simulink model "Observadores_Mimo19"  (R2023b)
settings: Solver=ode23t  StartTime=0.0  StopTime=5  MaxStep=1e-3  RelTol=1e-3
values from neighbouring files (symbols this model uses):
  Ac = reg.a    [Observdores_funcion_lqg.m]    (also in Observdores_pto_equilibrio.m)
  Ac_1 = [AL-BL*Kest-L*CL+L*DL*Kest, BL*Ki - L*DL*Ki ... (first row only)    [Observdores.m]
  Ac_2 = reg.a    [Observdores.m]    (also in Observdores_funcion_lqg.m; lqg_funcion.m)
  AL = double(subs(A,{a,b,c,d},{a1,b1,c1,d1}))    [Observdores.m]    (also in Observdores_funcion_lqg.m = double(subs(A,{x1,x2,x3,x4,u1,u2,u3,u4},{x10,x20,x30,x40,u10; Observdores_pto_equilibrio.m; Observdores_pto_equilibrio_discreto.m; Observdores_seguimiento_discreto.m)
  Bc = reg.b    [Observdores_funcion_lqg.m]    (also in Observdores_pto_equilibrio.m)
  Bc_1 = [-L ... (first row only)    [Observdores.m]
  Bc_2 = reg.b    [Observdores.m]    (also in Observdores_funcion_lqg.m; lqg_funcion.m)
  BL = double(subs(B,{a,b,c,d},{a1,b1,c1,d1}))    [Observdores.m]    (also in Observdores_funcion_lqg.m = double(subs(B,{x1,x2,x3,x4,u1,u2,u3,u4},{x10,x20,x30,x40,u10; Observdores_pto_equilibrio.m; Observdores_pto_equilibrio_discreto.m; Observdores_seguimiento_discreto.m)
  Cc = sys_d2.c    [Observdores.m]    (also in Observdores_funcion_lqg.m = reg.c; Observdores_pto_equilibrio.m = reg.c; Observdores_pto_equilibrio_discreto.m = -K)
  Cc_1 = [-Kest, Ki]    [Observdores.m]
  Cc_2 = reg.c    [Observdores.m]    (also in Observdores_funcion_lqg.m; lqg_funcion.m)
  Ccon = [-Kest Ki]    [Observdores_seguimiento_discreto.m]
  CL = [1 0 0 ... (first row only)    [Observdores.m]    (also in Observdores_funcion_lqg.m = [1 1 0 0; Observdores_pto_equilibrio.m; Observdores_pto_equilibrio_discreto.m; Observdores_seguimiento_discreto.m)
  Dc = reg.d    [Observdores_funcion_lqg.m]    (also in Observdores_pto_equilibrio.m; Observdores_pto_equilibrio_discreto.m = zeros(p,r))
  Dc_1 = zeros(p,r)    [Observdores.m]
  Dc_2 = reg.d    [Observdores.m]    (also in Observdores_funcion_lqg.m; lqg_funcion.m)
  Dcon = zeros(p,2*r)    [Observdores_seguimiento_discreto.m]
  DL = [0 0 0 ... (first row only)    [Observdores.m]    (also in Observdores_funcion_lqg.m = [0 0 0 0; Observdores_pto_equilibrio.m; Observdores_pto_equilibrio_discreto.m; Observdores_seguimiento_discreto.m)
  Gc = sys_d2.a    [Observdores.m]    (also in Observdores_pto_equilibrio.m = sys_c_dig.a; Observdores_pto_equilibrio_discreto.m = GL-HL*K-L*CL+L*DL*K)
  Gcon = [GL-HL*Kest-L*CL+L*DL*Kest, HL*Ki - L*DL*Ki ... (first row only)    [Observdores_seguimiento_discreto.m]
  GL = sysd.a    [Observdores_pto_equilibrio_discreto.m]    (also in Observdores_seguimiento_discreto.m)
  Hc = sys_c_dig.b    [Observdores_pto_equilibrio.m]    (also in Observdores_pto_equilibrio_discreto.m = L)
  Hcon = [zeros(n,r), L ... (first row only)    [Observdores_seguimiento_discreto.m]
  HL = sysd.b    [Observdores_pto_equilibrio_discreto.m]    (also in Observdores_seguimiento_discreto.m)
  K = place(Ahat,Bhat,delta)    [Observdores.m]
  Kest = K(:,1:n)    [Observdores.m]    (also in Observdores_seguimiento_discreto.m)
  Ki = -K(:,n+1:end)    [Observdores.m]    (also in Observdores_seguimiento_discreto.m)
  L = (place(AL',CL',delta))'    [Observdores.m]    (also in Observdores_pto_equilibrio.m; Observdores_pto_equilibrio_discreto.m = place(GL',CL',pol_obv_d)'; Observdores_seguimiento_discreto.m = place(GL',CL',pol_obv_d)')
  sys_d1 = c2d(sys_c1,Tm)    [Observdores.m]
  sys_d2 = c2d(sys_c2,Tm)    [Observdores.m]
  Tm = 0.02    [Observdores.m]    (also in Observdores_pto_equilibrio.m; Observdores_pto_equilibrio_discreto.m = 0.05; Observdores_seguimiento_discreto.m = 0.05)
  u10 = (a1*x20 + b1*x10^2)/u20    [Observdores.m]    (also in Observdores_funcion_lqg.m = 1; Observdores_pto_equilibrio.m; Observdores_pto_equilibrio_discreto.m; Observdores_seguimiento_discreto.m)
  u20 = sqrt(c1*x30*x20)    [Observdores.m]    (also in Observdores_funcion_lqg.m = sqrt(x30*x20); Observdores_pto_equilibrio.m; Observdores_pto_equilibrio_discreto.m; Observdores_seguimiento_discreto.m)
  u30 = (d1*x30 - u10)/x10    [Observdores.m]    (also in Observdores_funcion_lqg.m = (x20 + x10^2 - u20^2)/u10; Observdores_pto_equilibrio.m; Observdores_pto_equilibrio_discreto.m; Observdores_seguimiento_discreto.m)
  x10 = 2    [Observdores.m]    (also in Observdores_funcion_lqg.m; Observdores_pto_equilibrio.m; Observdores_pto_equilibrio_discreto.m; Observdores_seguimiento_discreto.m)
  x20 = 4    [Observdores.m]    (also in Observdores_funcion_lqg.m = 8; Observdores_pto_equilibrio.m; Observdores_pto_equilibrio_discreto.m; Observdores_seguimiento_discreto.m)
  x30 = 4    [Observdores.m]    (also in Observdores_funcion_lqg.m = 2; Observdores_pto_equilibrio.m; Observdores_pto_equilibrio_discreto.m; Observdores_seguimiento_discreto.m)
  xini = [0.5; -0.3; -0.7; 0.9]    [Observdores_funcion_lqg.m]    (also in Observdores_pto_equilibrio.m = [0.2; -0.3; -0.4]; Observdores_pto_equilibrio_discreto.m = [0.2; -0.3; -0.4])
undefined symbols (not defined in the file or in its folder): magnitude
libraries: simulink x22
(part 1 of 3)
settings Model: Creator=B12
settings SolverCC: AlgebraicLoopSolver=TrustRegion
settings DataIOCC: ReturnWorkspaceOutputs=off
settings DebuggingCC: UnconnectedInputMsg=warning  UnconnectedOutputMsg=warning  UnconnectedLineMsg=warning  ArithmeticOperatorsInVariantConditions=warning
settings ModelReferenceCC: EnableRefExpFcnMdlSchedulingChecks=on
settings SFSimCC: CustomCodeUndefinedFunction=UseInterfaceOnly

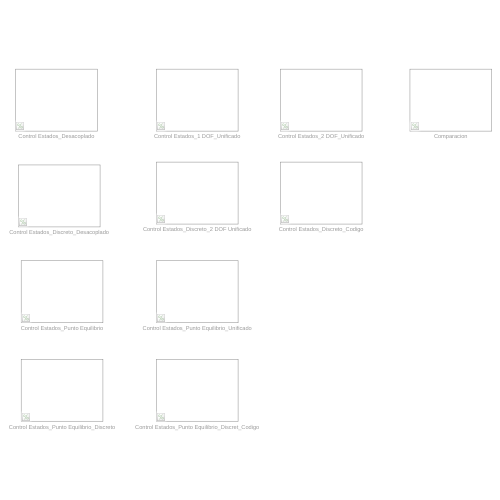
[thumbnail: Simulink's stored preview of the top-level diagram]
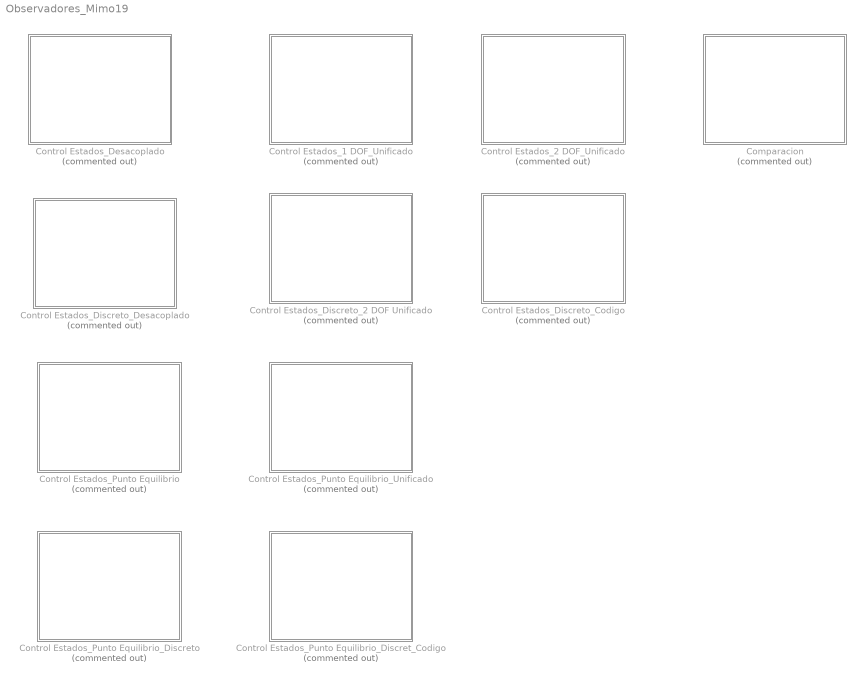
== system Observadores_Mimo19 ==
  Comparacion : Subsystem  Commented=on
  Control Estados_1 DOF_Unificado : Subsystem  Commented=on
  Control Estados_2 DOF_Unificado : Subsystem  Commented=on
  Control Estados_Desacoplado : Subsystem  Commented=on
  Control Estados_Discreto_2 DOF Unificado : Subsystem  Commented=on
  Control Estados_Discreto_Codigo : Subsystem  Commented=on
  Control Estados_Discreto_Desacoplado : Subsystem  Commented=on
  Control Estados_Punto Equilibrio : Subsystem  Commented=on
  Control Estados_Punto Equilibrio_Discret_Codigo : Subsystem  Commented=on
  Control Estados_Punto Equilibrio_Discreto : Subsystem  Commented=on
  Control Estados_Punto Equilibrio_Unificado : Subsystem  Commented=on

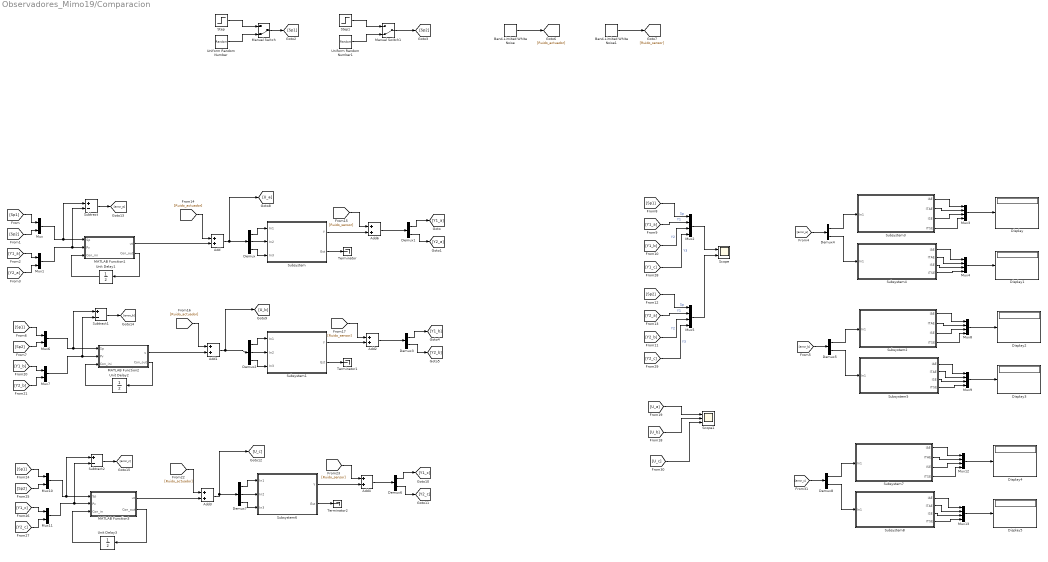
== system Observadores_Mimo19/Comparacion ==
  Add{,1..4,6} (6 alike) : Sum
  Band-Limited White Noise : simulink/Sources/Band-Limited White Noise  Cov=[1e-10 1e-10 1e-10 ]  Ts=0.001  seed=[23341]
  Band-Limited White Noise1 : simulink/Sources/Band-Limited White Noise  Cov=[1e-10 1e-10 ]  Ts=0.001  seed=[23341]
  Demux : Demux  Outputs=3
  Demux{1,3..6,8} (6 alike) : Demux  Outputs=2
  Demux2 : Demux  Outputs=3
  Demux7 : Demux  Outputs=3
  Display{,1..5} (6 alike) : Display
  MATLAB Function1 : MATLAB Function  TreatAsAtomicUnit=on
  MATLAB Function2 : MATLAB Function  TreatAsAtomicUnit=on
  MATLAB Function3 : MATLAB Function  TreatAsAtomicUnit=on
  Manual Switch : ManualSwitch  CurrentSetting=0
  Manual Switch1 : ManualSwitch  CurrentSetting=0
  Mux{,1,6..7,10..11} (6 alike) : Mux  Inputs=2
  Mux{2..5,8..9,12..13} (8 alike) : Mux
  Scope : Scope  NumInputPorts=2
  Scope1 : Scope  NumInputPorts=3
  Step : Step  Time=0  After=0.5  SampleTime=0
  Step1 : Step  Time=0  After=0.5  SampleTime=0
  Subsystem : Subsystem
  Subsystem1 : Subsystem
  Subsystem2 : Subsystem
  Subsystem3 : Subsystem
  Subsystem4 : Subsystem
  Subsystem5 : Subsystem
  Subsystem6 : Subsystem
  Subsystem7 : Subsystem
  Subsystem8 : Subsystem
  Subtract : Sum  Inputs=+-
  Subtract1 : Sum  Inputs=+-
  Subtract2 : Sum  Inputs=+-
  Terminator : Terminator
  Terminator1 : Terminator
  Terminator2 : Terminator
  Uniform Random Number : UniformRandomNumber  Minimum=-0.5  Maximum=0.5  SampleTime=4
  Uniform Random Number1 : UniformRandomNumber  Minimum=-0.5  Maximum=0.5  Seed=6  SampleTime=7
  Unit Delay1 : UnitDelay  InitialCondition=zeros(8,1)  SampleTime=Tm  HasFrameUpgradeWarning=on
  Unit Delay2 : UnitDelay  InitialCondition=zeros(8,1)  SampleTime=Tm  HasFrameUpgradeWarning=on
  Unit Delay3 : UnitDelay  InitialCondition=zeros(8,1)  SampleTime=Tm  HasFrameUpgradeWarning=on
  wires:
  [Sp2] -> Mux5/1  "Sp"
  [Y1_a] -> Mux2/2  "Y1"
  [U_a] -> Scope1/1
  [Y2_a] -> Mux5/2  "Y1"
  [U_b] -> Scope1/2
  [Y2_b] -> Mux5/3  "Y2"
  Mux2/1 -> Scope/1
  [Sp1] -> Mux2/1  "Sp"
  [Y1_b] -> Mux2/3  "Y2"
  Mux5/1 -> Scope/2
  Mux3/1 -> Display/1
  Demux4/2 -> Subsystem4/1(In1)
  Demux4/1 -> Subsystem3/1(In1)
  Mux4/1 -> Display1/1
  [error_a] -> Demux4/1
  Subsystem4/1(IAE) -> Mux4/1
  Subsystem4/2(ITAE) -> Mux4/2
  Subsystem4/3(ISE) -> Mux4/3
  Subsystem4/4(ITSE) -> Mux4/4
  Subsystem3/1(IAE) -> Mux3/1
  Subsystem3/2(ITAE) -> Mux3/2
  Subsystem3/3(ISE) -> Mux3/3
  Subsystem3/4(ITSE) -> Mux3/4
  Subsystem2/1(IAE) -> Mux8/1
  Subsystem2/2(ITAE) -> Mux8/2
  [error_b] -> Demux5/1
  Mux9/1 -> Display3/1
  Demux5/2 -> Subsystem5/1(In1)
  Mux8/1 -> Display2/1
  Subsystem2/4(ITSE) -> Mux8/4
  Subsystem5/4(ITSE) -> Mux9/4
  Subsystem5/1(IAE) -> Mux9/1
  Demux5/1 -> Subsystem2/1(In1)
  Subsystem5/2(ITAE) -> Mux9/2
  Subsystem2/3(ISE) -> Mux8/3
  Subsystem5/3(ISE) -> Mux9/3
  [Y1_c] -> Mux2/4  "Y3"
  [Y2_c] -> Mux5/4  "Y3"
  [U_c] -> Scope1/3
  Subsystem7/4(ITSE) -> Mux12/4
  Subsystem8/4(ITSE) -> Mux13/4
  Mux12/1 -> Display4/1
  Demux8/2 -> Subsystem8/1(In1)
  [error_c] -> Demux8/1
  Subsystem8/1(IAE) -> Mux13/1
  Subsystem8/2(ITAE) -> Mux13/2
  Subsystem8/3(ISE) -> Mux13/3
  Subsystem7/1(IAE) -> Mux12/1
  Mux13/1 -> Display5/1
  Subsystem7/2(ITAE) -> Mux12/2
  Subsystem7/3(ISE) -> Mux12/3
  Demux8/1 -> Subsystem7/1(In1)
  Band-Limited White Noise1/1 -> [Ruido_sensor]
  Uniform Random Number1/1 -> Manual Switch1/2
  Band-Limited White Noise/1 -> [Ruido_actuador]
  Manual Switch1/1 -> [Sp2]
  Manual Switch/1 -> [Sp1]
  Uniform Random Number/1 -> Manual Switch/2
  Step/1 -> Manual Switch/1
  Step1/1 -> Manual Switch1/1
  Demux/3 -> Subsystem/3(In3)
  Add/1 -> Demux/1, [U_a]
  Demux/2 -> Subsystem/2(In2)
  Unit Delay1/1 -> MATLAB Function1/3(Con_ini)
  [Y2_a] -> Mux1/2
  Demux/1 -> Subsystem/1(In1)
  [Y1_a] -> Mux1/1
  Subsystem/2(Est) -> Terminator/1
  Subsystem/1(Y) -> Add6/2
  [Ruido_actuador] -> Add/1
  Mux/1 -> Subtract/1, MATLAB Function1/1(Sp)
  MATLAB Function1/2(Con_out) -> Unit Delay1/1
  [Sp2] -> Mux/2
  Add6/1 -> Demux1/1
  Demux1/1 -> [Y1_a]
  Mux1/1 -> Subtract/2, MATLAB Function1/2(Pv)
  [Ruido_sensor] -> Add6/1
  Demux1/2 -> [Y2_a]
  [Sp1] -> Mux/1
  MATLAB Function1/1(ut) -> Add/2
  Subsystem1/2(Est) -> Terminator1/1
  Demux2/1 -> Subsystem1/1(In1)
  Demux3/2 -> [Y2_b]
  Unit Delay2/1 -> MATLAB Function2/3(Con_ini)
  Demux2/3 -> Subsystem1/3(In3)
  MATLAB Function2/2(Con_out) -> Unit Delay2/1
  Demux3/1 -> [Y1_b]
  Mux7/1 -> Subtract1/2, MATLAB Function2/2(Pv)
  [Ruido_actuador] -> Add1/1
  [Ruido_sensor] -> Add2/1
  [Y2_b] -> Mux7/2
  Add1/1 -> [U_b], Demux2/1
  [Sp1] -> Mux6/1
  Subsystem1/1(Y) -> Add2/2
  Demux2/2 -> Subsystem1/2(In2)
  Mux6/1 -> Subtract1/1, MATLAB Function2/1(Sp)
  [Sp2] -> Mux6/2
  [Y1_b] -> Mux7/1
  Add2/1 -> Demux3/1
  MATLAB Function2/1(u) -> Add1/2
  Subsystem6/2(Est) -> Terminator2/1
  [Sp2] -> Mux10/2
  Add4/1 -> Demux6/1
  Demux7/1 -> Subsystem6/1(In1)
  Demux6/1 -> [Y1_c]
  [Y1_c] -> Mux11/1
  Subsystem6/1(Y) -> Add4/2
  Demux7/3 -> Subsystem6/3(In3)
  Mux11/1 -> Subtract2/2, MATLAB Function3/2(Pv)
  Mux10/1 -> Subtract2/1, MATLAB Function3/1(Sp)
  MATLAB Function3/2(Con_out) -> Unit Delay3/1
  [Sp1] -> Mux10/1
  Add3/1 -> Demux7/1, [U_c]
  Demux6/2 -> [Y2_c]
  [Y2_c] -> Mux11/2
  [Ruido_sensor] -> Add4/1
  MATLAB Function3/1(ut) -> Add3/2
  Unit Delay3/1 -> MATLAB Function3/3(Con_in)
  Demux7/2 -> Subsystem6/2(In2)
  [Ruido_actuador] -> Add3/1
  Subtract/1 -> [error_a]
  Subtract1/1 -> [error_b]
  Subtract2/1 -> [error_c]

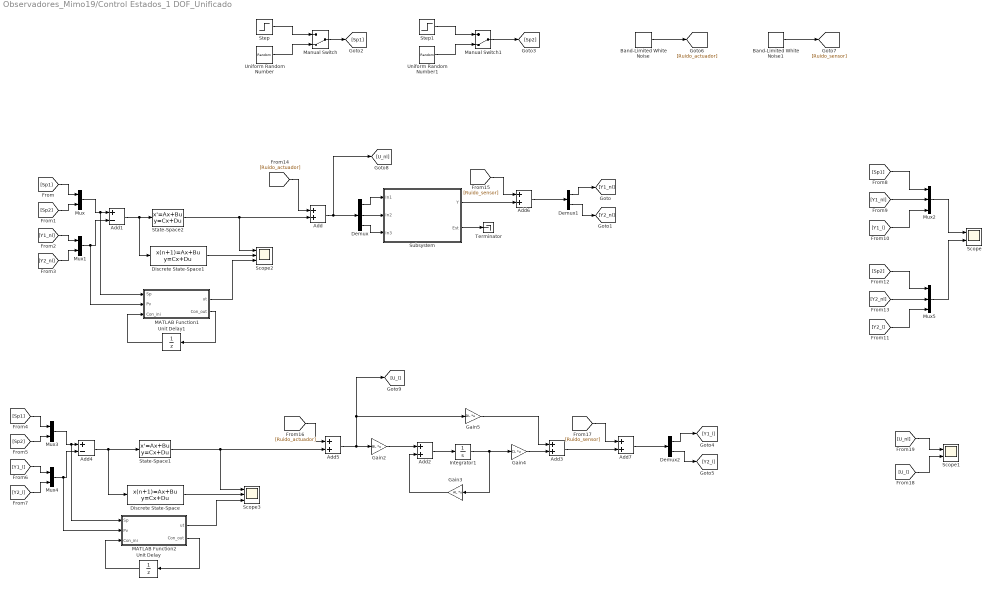
== system Observadores_Mimo19/Control Estados_1 DOF_Unificado ==
  Add{,2..3,5..7} (6 alike) : Sum
  Add1 : Sum  Inputs=+-
  Add4 : Sum  Inputs=+-
  Band-Limited White Noise : simulink/Sources/Band-Limited White Noise  Cov=[1e-10 1e-10 1e-10 ]  Ts=0.001  seed=[23341]
  Band-Limited White Noise1 : simulink/Sources/Band-Limited White Noise  Cov=[1e-10 1e-10 ]  Ts=0.001  seed=[23341]
  Demux : Demux  Outputs=3
  Demux1 : Demux  Outputs=2
  Demux2 : Demux  Outputs=2
  Discrete State-Space : DiscreteStateSpace  A=sys_d1.a  B=sys_d1.b  C=sys_d1.c  D=sys_d1.d  SampleTime=Tm
  Discrete State-Space1 : DiscreteStateSpace  A=sys_d1.a  B=sys_d1.b  C=sys_d1.c  D=sys_d1.d  SampleTime=Tm
  Gain2 : Gain  Gain=BL  Multiplication=Matrix(K*u)
  Gain3 : Gain  Gain=AL  Multiplication=Matrix(K*u)
  Gain4 : Gain  Gain=CL  Multiplication=Matrix(K*u)
  Gain5 : Gain  Gain=DL  Multiplication=Matrix(K*u)
  Integrator1 : Integrator
  MATLAB Function1 : MATLAB Function  TreatAsAtomicUnit=on
  MATLAB Function2 : MATLAB Function  TreatAsAtomicUnit=on
  Manual Switch : ManualSwitch  CurrentSetting=0
  Manual Switch1 : ManualSwitch  CurrentSetting=0
  Mux{,1,3..4} (4 alike) : Mux  Inputs=2
  Mux2 : Mux  Inputs=3
  Mux5 : Mux  Inputs=3
  Scope : Scope  NumInputPorts=2
  Scope1 : Scope  NumInputPorts=2
  Scope2 : Scope  NumInputPorts=3
  Scope3 : Scope  NumInputPorts=3
  State-Space1 : StateSpace  A=Ac_1  B=Bc_1  C=Cc_1  D=Dc_1  InitialCondition=0
  State-Space2 : StateSpace  A=Ac_1  B=Bc_1  C=Cc_1  D=Dc_1  InitialCondition=0
  Step : Step  Time=0  After=0.5  SampleTime=0
  Step1 : Step  Time=0  After=0.5  SampleTime=0
  Subsystem : Subsystem
  Terminator : Terminator
  Uniform Random Number : UniformRandomNumber  Minimum=-0.5  Maximum=0.5  SampleTime=4
  Uniform Random Number1 : UniformRandomNumber  Minimum=-0.5  Maximum=0.5  Seed=6  SampleTime=7
  Unit Delay : UnitDelay  InitialCondition=zeros(8,1)  SampleTime=Tm  HasFrameUpgradeWarning=on
  Unit Delay1 : UnitDelay  InitialCondition=zeros(8,1)  SampleTime=Tm  HasFrameUpgradeWarning=on
  wires:
  [Sp2] -> Mux5/1
  Add7/1 -> Demux2/1
  Mux/1 -> MATLAB Function1/1(Sp), Add1/1
  [Ruido_actuador] -> Add/1
  Add6/1 -> Demux1/1
  [Y1_nl] -> Mux2/2
  [U_nl] -> Scope1/1
  Add5/1 -> [U_l], Gain5/1, Gain2/1
  [Ruido_sensor] -> Add6/1
  Gain2/1 -> Add2/1
  Gain5/1 -> Add3/1
  [Ruido_actuador] -> Add5/1
  [Y2_nl] -> Mux5/2
  Demux1/2 -> [Y2_nl]
  [Sp1] -> Mux/1
  [Y1_nl] -> Mux1/1
  [U_l] -> Scope1/2
  [Y2_l] -> Mux5/3
  Mux1/1 -> MATLAB Function1/2(Pv), Add1/2
  [Ruido_sensor] -> Add7/1
  Gain4/1 -> Add3/2
  Mux4/1 -> MATLAB Function2/2(Pv), Add4/2
  [Sp2] -> Mux/2
  [Sp1] -> Mux3/1
  Integrator1/1 -> Gain4/1, Gain3/1
  [Sp2] -> Mux3/2
  Demux2/1 -> [Y1_l]
  Gain3/1 -> Add2/2
  [Y2_nl] -> Mux1/2
  Mux2/1 -> Scope/1
  Demux1/1 -> [Y1_nl]
  [Sp1] -> Mux2/1
  Demux2/2 -> [Y2_l]
  [Y1_l] -> Mux4/1
  Mux3/1 -> MATLAB Function2/1(Sp), Add4/1
  [Y2_l] -> Mux4/2
  [Y1_l] -> Mux2/3
  Add2/1 -> Integrator1/1
  Mux5/1 -> Scope/2
  Add3/1 -> Add7/2
  Add4/1 -> Discrete State-Space/1, State-Space1/1
  State-Space1/1 -> Add5/2, Scope3/1
  Add1/1 -> Discrete State-Space1/1, State-Space2/1
  MATLAB Function2/2(Con_out) -> Unit Delay/1
  Unit Delay/1 -> MATLAB Function2/3(Con_ini)
  Unit Delay1/1 -> MATLAB Function1/3(Con_ini)
  MATLAB Function1/2(Con_out) -> Unit Delay1/1
  State-Space2/1 -> Add/2, Scope2/1
  Discrete State-Space1/1 -> Scope2/2
  MATLAB Function1/1(ut) -> Scope2/3
  Add/1 -> Demux/1, [U_nl]
  Demux/3 -> Subsystem/3(In3)
  Demux/2 -> Subsystem/2(In2)
  Demux/1 -> Subsystem/1(In1)
  Subsystem/1(Y) -> Add6/2
  Subsystem/2(Est) -> Terminator/1
  Discrete State-Space/1 -> Scope3/2
  MATLAB Function2/1(ut) -> Scope3/3
  Band-Limited White Noise/1 -> [Ruido_actuador]
  Uniform Random Number/1 -> Manual Switch/2
  Manual Switch/1 -> [Sp1]
  Uniform Random Number1/1 -> Manual Switch1/2
  Step/1 -> Manual Switch/1
  Step1/1 -> Manual Switch1/1
  Band-Limited White Noise1/1 -> [Ruido_sensor]
  Manual Switch1/1 -> [Sp2]

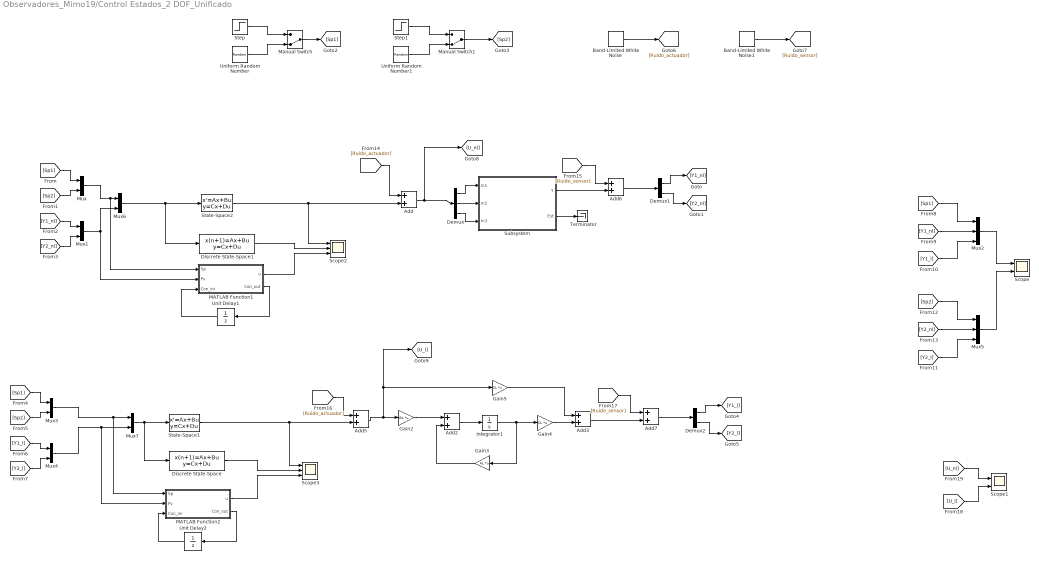
== system Observadores_Mimo19/Control Estados_2 DOF_Unificado ==
  Add{,2..3,5..7} (6 alike) : Sum
  Band-Limited White Noise : simulink/Sources/Band-Limited White Noise  Cov=[1e-10 1e-10 1e-10 ]  Ts=0.001  seed=[23341]
  Band-Limited White Noise1 : simulink/Sources/Band-Limited White Noise  Cov=[1e-10 1e-10 ]  Ts=0.001  seed=[23341]
  Demux : Demux  Outputs=3
  Demux1 : Demux  Outputs=2
  Demux2 : Demux  Outputs=2
  Discrete State-Space : DiscreteStateSpace  A=sys_d2.a  B=sys_d2.b  C=sys_d2.c  D=sys_d2.d  SampleTime=Tm
  Discrete State-Space1 : DiscreteStateSpace  A=sys_d2.a  B=sys_d2.b  C=sys_d2.c  D=sys_d2.d  SampleTime=Tm
  Gain2 : Gain  Gain=BL  Multiplication=Matrix(K*u)
  Gain3 : Gain  Gain=AL  Multiplication=Matrix(K*u)
  Gain4 : Gain  Gain=CL  Multiplication=Matrix(K*u)
  Gain5 : Gain  Gain=DL  Multiplication=Matrix(K*u)
  Integrator1 : Integrator
  MATLAB Function1 : MATLAB Function  TreatAsAtomicUnit=on
  MATLAB Function2 : MATLAB Function  TreatAsAtomicUnit=on
  Manual Switch : ManualSwitch  CurrentSetting=0
  Manual Switch1 : ManualSwitch  CurrentSetting=0
  Mux{,1,3..4,6..7} (6 alike) : Mux  Inputs=2
  Mux2 : Mux  Inputs=3
  Mux5 : Mux  Inputs=3
  Scope : Scope  NumInputPorts=2
  Scope1 : Scope  NumInputPorts=2
  Scope2 : Scope  NumInputPorts=3
  Scope3 : Scope  NumInputPorts=3
  State-Space1 : StateSpace  A=Ac_2  B=Bc_2  C=Cc_2  D=Dc_2  InitialCondition=0
  State-Space2 : StateSpace  A=Ac_2  B=Bc_2  C=Cc_2  D=Dc_2  InitialCondition=0
  Step : Step  Time=0  After=0.5  SampleTime=0
  Step1 : Step  Time=0  After=0.5  SampleTime=0
  Subsystem : Subsystem
  Terminator : Terminator
  Uniform Random Number : UniformRandomNumber  Minimum=-0.5  Maximum=0.5  SampleTime=4
  Uniform Random Number1 : UniformRandomNumber  Minimum=-0.5  Maximum=0.5  Seed=6  SampleTime=7
  Unit Delay1 : UnitDelay  InitialCondition=zeros(8,1)  SampleTime=Tm  HasFrameUpgradeWarning=on
  Unit Delay2 : UnitDelay  InitialCondition=zeros(8,1)  SampleTime=Tm  HasFrameUpgradeWarning=on
  wires:
  [Sp2] -> Mux5/1
  Add7/1 -> Demux2/1
  Mux/1 -> MATLAB Function1/1(Sp), Mux6/1
  Add/1 -> [U_nl], Demux/1
  [Ruido_actuador] -> Add/1
  Add6/1 -> Demux1/1
  [Y1_nl] -> Mux2/2
  [U_nl] -> Scope1/1
  Add5/1 -> [U_l], Gain5/1, Gain2/1
  [Ruido_sensor] -> Add6/1
  Gain2/1 -> Add2/1
  Gain5/1 -> Add3/1
  [Ruido_actuador] -> Add5/1
  [Y2_nl] -> Mux5/2
  Demux1/2 -> [Y2_nl]
  [Sp1] -> Mux/1
  [Y1_nl] -> Mux1/1
  [U_l] -> Scope1/2
  [Y2_l] -> Mux5/3
  Mux1/1 -> MATLAB Function1/2(Pv), Mux6/2
  [Ruido_sensor] -> Add7/1
  Gain4/1 -> Add3/2
  [Sp2] -> Mux/2
  [Sp1] -> Mux3/1
  Integrator1/1 -> Gain4/1, Gain3/1
  [Sp2] -> Mux3/2
  Demux2/1 -> [Y1_l]
  Gain3/1 -> Add2/2
  [Y2_nl] -> Mux1/2
  Mux2/1 -> Scope/1
  Demux1/1 -> [Y1_nl]
  [Sp1] -> Mux2/1
  Demux2/2 -> [Y2_l]
  [Y1_l] -> Mux4/1
  [Y2_l] -> Mux4/2
  [Y1_l] -> Mux2/3
  Add2/1 -> Integrator1/1
  Mux5/1 -> Scope/2
  Add3/1 -> Add7/2
  Mux3/1 -> MATLAB Function2/1(Sp), Mux7/1
  Mux4/1 -> MATLAB Function2/2(Pv), Mux7/2
  Mux7/1 -> State-Space1/1, Discrete State-Space/1
  Mux6/1 -> Discrete State-Space1/1, State-Space2/1
  Unit Delay1/1 -> MATLAB Function1/3(Con_ini)
  MATLAB Function1/2(Con_out) -> Unit Delay1/1
  State-Space2/1 -> Scope2/1, Add/2
  MATLAB Function2/2(Con_out) -> Unit Delay2/1
  Unit Delay2/1 -> MATLAB Function2/3(Con_ini)
  Demux/3 -> Subsystem/3(In3)
  Subsystem/2(Est) -> Terminator/1
  Demux/1 -> Subsystem/1(In1)
  Demux/2 -> Subsystem/2(In2)
  Subsystem/1(Y) -> Add6/2
  Discrete State-Space1/1 -> Scope2/2
  MATLAB Function1/1(u) -> Scope2/3
  Manual Switch/1 -> [Sp1]
  Manual Switch1/1 -> [Sp2]
  Band-Limited White Noise1/1 -> [Ruido_sensor]
  Step1/1 -> Manual Switch1/1
  Band-Limited White Noise/1 -> [Ruido_actuador]
  Step/1 -> Manual Switch/1
  Uniform Random Number/1 -> Manual Switch/2
  Uniform Random Number1/1 -> Manual Switch1/2
  State-Space1/1 -> Scope3/1, Add5/2
  Discrete State-Space/1 -> Scope3/2
  MATLAB Function2/1(u) -> Scope3/3

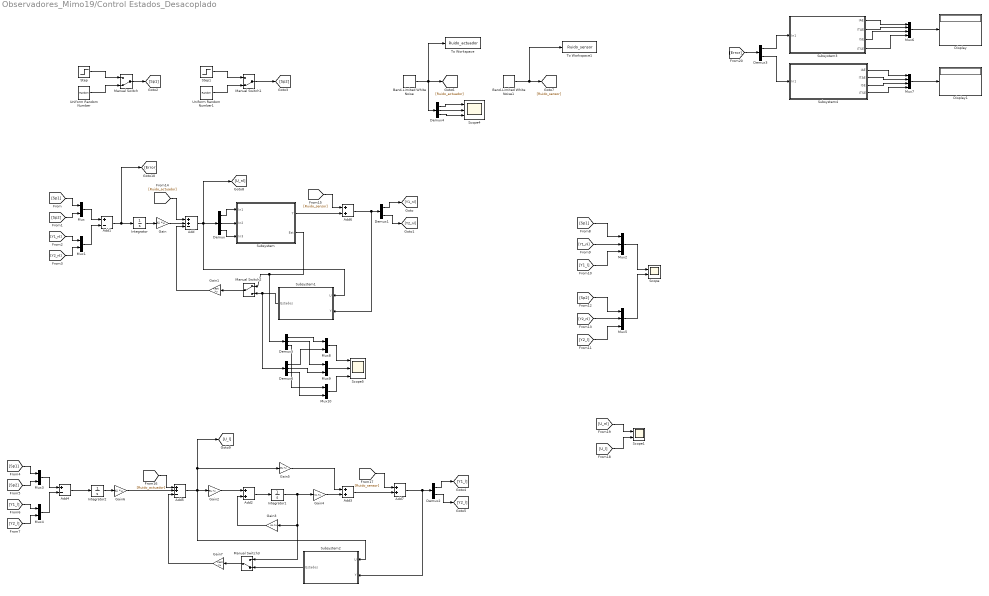
== system Observadores_Mimo19/Control Estados_Desacoplado ==
  Add : Sum  Inputs=++-
  Add1 : Sum  Inputs=+-
  Add{2..3,6..7} (4 alike) : Sum
  Add4 : Sum  Inputs=+-
  Add5 : Sum  Inputs=++-
  Band-Limited White Noise : simulink/Sources/Band-Limited White Noise  Cov=[1e-10 1e-10 1e-10 ]  Ts=0.001  seed=[23341]
  Band-Limited White Noise1 : simulink/Sources/Band-Limited White Noise  Cov=[1e-10 1e-10 ]  Ts=0.001  seed=[23341]
  Demux{,4..6} (4 alike) : Demux  Outputs=3
  Demux1 : Demux  Outputs=2
  Demux2 : Demux  Outputs=2
  Demux3 : Demux  Outputs=2
  Display : Display
  Display1 : Display
  Gain : Gain  Gain=Ki  Multiplication=Matrix(K*u)
  Gain1 : Gain  Gain=Kest  Multiplication=Matrix(K*u)
  Gain2 : Gain  Gain=BL  Multiplication=Matrix(K*u)
  Gain3 : Gain  Gain=AL  Multiplication=Matrix(K*u)
  Gain4 : Gain  Gain=CL  Multiplication=Matrix(K*u)
  Gain5 : Gain  Gain=DL  Multiplication=Matrix(K*u)
  Gain6 : Gain  Gain=Ki  Multiplication=Matrix(K*u)
  Gain7 : Gain  Gain=Kest  Multiplication=Matrix(K*u)
  Integrator : Integrator
  Integrator1 : Integrator
  Integrator2 : Integrator
  Manual Switch : ManualSwitch  CurrentSetting=0
  Manual Switch1 : ManualSwitch  CurrentSetting=0
  Manual Switch2 : ManualSwitch
  Manual Switch3 : ManualSwitch  CurrentSetting=0
  Mux{,1,3..4,8..10} (7 alike) : Mux  Inputs=2
  Mux2 : Mux  Inputs=3
  Mux5 : Mux  Inputs=3
  Mux6 : Mux
  Mux7 : Mux
  Scope : Scope  NumInputPorts=2
  Scope1 : Scope  NumInputPorts=2
  Scope4 : Scope  NumInputPorts=3
  Scope5 : Scope  NumInputPorts=3
  Step : Step  Time=0  After=0.5  SampleTime=0
  Step1 : Step  Time=0  After=0.5  SampleTime=0
  Subsystem : Subsystem
  Subsystem1 : Subsystem
  Subsystem2 : Subsystem
  Subsystem3 : Subsystem
  Subsystem4 : Subsystem
  To Workspace : ToWorkspace  VariableName=Ruido_actuador  SampleTime=-1
  To Workspace1 : ToWorkspace  VariableName=Ruido_sensor  SampleTime=-1
  Uniform Random Number : UniformRandomNumber  Minimum=-0.5  Maximum=0.5  SampleTime=4
  Uniform Random Number1 : UniformRandomNumber  Minimum=-0.5  Maximum=0.5  Seed=6  SampleTime=7
  wires:
  Gain/1 -> Add/2
  Subsystem2/1(Estados) -> Manual Switch3/2
  [Sp2] -> Mux5/1
  Add7/1 -> Subsystem2/2(Y), Demux2/1
  Mux/1 -> Add1/1
  Add/1 -> Subsystem1/1(U), [U_nl], Demux/1
  [Ruido_actuador] -> Add/1
  Add6/1 -> Subsystem1/2(Y), Demux1/1
  [Y1_nl] -> Mux2/2
  [U_nl] -> Scope1/1
  Gain1/1 -> Add/3
  Gain6/1 -> Add5/2
  Add5/1 -> Subsystem2/1(U), [U_l], Gain5/1, Gain2/1
  [Ruido_sensor] -> Add6/1
  Gain2/1 -> Add2/1
  Gain5/1 -> Add3/1
  [Ruido_actuador] -> Add5/1
  Manual Switch1/1 -> [Sp2]
  [Y2_nl] -> Mux5/2
  Band-Limited White Noise1/1 -> To Workspace1/1, [Ruido_sensor]
  Demux1/2 -> [Y2_nl]
  [Sp1] -> Mux/1
  [Y1_nl] -> Mux1/1
  Subsystem1/1(Estados) -> Demux6/1, Manual Switch2/2
  [U_l] -> Scope1/2
  Subsystem/1(Y) -> Add6/2
  Step1/1 -> Manual Switch1/1
  Integrator2/1 -> Gain6/1
  Gain7/1 -> Add5/3
  [Y2_l] -> Mux5/3
  Manual Switch3/1 -> Gain7/1
  Mux1/1 -> Add1/2
  [Ruido_sensor] -> Add7/1
  Gain4/1 -> Add3/2
  Demux/3 -> Subsystem/3(In3)
  Add1/1 -> [Error], Integrator/1
  Subsystem/2(Est) -> Demux5/1, Manual Switch2/1
  Integrator/1 -> Gain/1
  Mux4/1 -> Add4/2
  [Sp2] -> Mux/2
  Demux/2 -> Subsystem/2(In2)
  [Sp1] -> Mux3/1
  Integrator1/1 -> Gain4/1, Gain3/1, Manual Switch3/1
  [Sp2] -> Mux3/2
  Uniform Random Number1/1 -> Manual Switch1/2
  Manual Switch/1 -> [Sp1]
  Demux2/1 -> [Y1_l]
  Gain3/1 -> Add2/2
  Step/1 -> Manual Switch/1
  [Y2_nl] -> Mux1/2
  Mux2/1 -> Scope/1
  Demux/1 -> Subsystem/1(In1)
  Demux1/1 -> [Y1_nl]
  [Sp1] -> Mux2/1
  Demux2/2 -> [Y2_l]
  [Y1_l] -> Mux4/1
  Mux3/1 -> Add4/1
  [Y2_l] -> Mux4/2
  Uniform Random Number/1 -> Manual Switch/2
  [Y1_l] -> Mux2/3
  Manual Switch2/1 -> Gain1/1
  Add2/1 -> Integrator1/1
  Mux5/1 -> Scope/2
  Add4/1 -> Integrator2/1
  Add3/1 -> Add7/2
  Band-Limited White Noise/1 -> Demux4/1, To Workspace/1, [Ruido_actuador]
  [Error] -> Demux3/1
  Demux3/1 -> Subsystem3/1(In1)
  Demux3/2 -> Subsystem4/1(In1)
  Subsystem3/1(IAE) -> Mux6/1
  Subsystem3/2(ITAE) -> Mux6/2
  Subsystem4/1(IAE) -> Mux7/1
  Subsystem4/2(ITAE) -> Mux7/2
  Subsystem4/3(ISE) -> Mux7/3
  Subsystem4/4(ITSE) -> Mux7/4
  Mux6/1 -> Display/1
  Mux7/1 -> Display1/1
  Demux4/1 -> Scope4/1
  Demux4/2 -> Scope4/2
  Demux4/3 -> Scope4/3
  Demux5/1 -> Mux8/1
  Demux6/1 -> Mux8/2
  Demux6/2 -> Mux9/2
  Demux5/2 -> Mux9/1
  Demux5/3 -> Mux10/1
  Demux6/3 -> Mux10/2
  Mux8/1 -> Scope5/1
  Mux9/1 -> Scope5/2
  Mux10/1 -> Scope5/3
  Subsystem3/3(ISE) -> Mux6/3
  Subsystem3/4(ITSE) -> Mux6/4

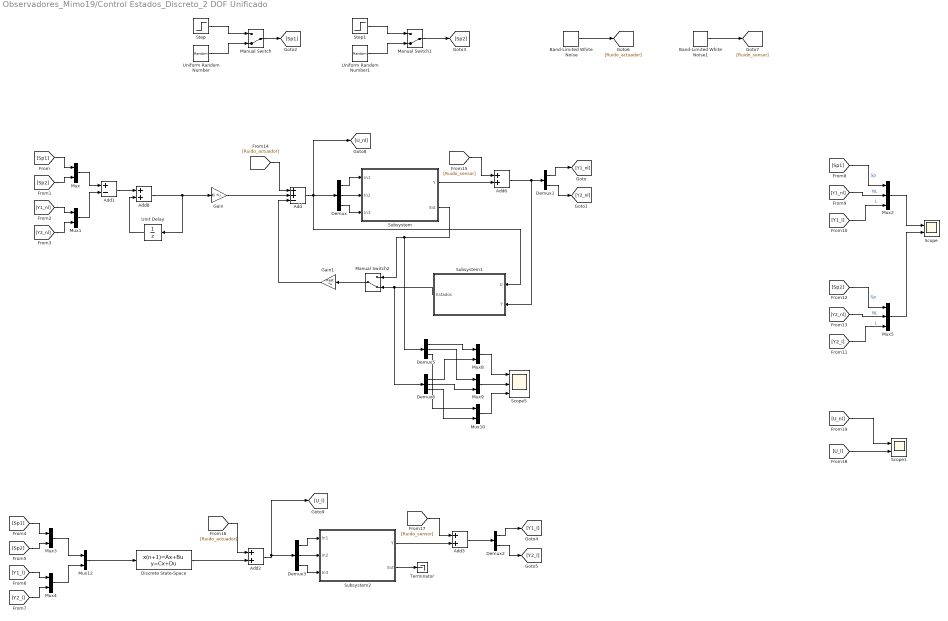
== system Observadores_Mimo19/Control Estados_Discreto_2 DOF Unificado ==
  Add : Sum  Inputs=++-
  Add1 : Sum  Inputs=+-
  Add{2..3,6,8} (4 alike) : Sum
  Band-Limited White Noise : simulink/Sources/Band-Limited White Noise  Cov=[1e-10 1e-10 1e-10 ]  Ts=0.001  seed=[23341]
  Band-Limited White Noise1 : simulink/Sources/Band-Limited White Noise  Cov=[1e-10 1e-10 ]  Ts=0.001  seed=[23341]
  Demux{,3,5..6} (4 alike) : Demux  Outputs=3
  Demux1 : Demux  Outputs=2
  Demux2 : Demux  Outputs=2
  Discrete State-Space : DiscreteStateSpace  A=Gcon  B=Hcon  C=Ccon  D=Dcon  SampleTime=Tm
  Gain : Gain  Gain=Ki  Multiplication=Matrix(K*u)
  Gain1 : Gain  Gain=Kest  Multiplication=Matrix(K*u)
  Manual Switch : ManualSwitch  CurrentSetting=0
  Manual Switch1 : ManualSwitch  CurrentSetting=0
  Manual Switch2 : ManualSwitch  CurrentSetting=0
  Mux{,1,3..4,8..10,12} (8 alike) : Mux  Inputs=2
  Mux2 : Mux  Inputs=3
  Mux5 : Mux  Inputs=3
  Scope : Scope  NumInputPorts=2
  Scope1 : Scope  NumInputPorts=2
  Scope5 : Scope  NumInputPorts=3
  Step : Step  Time=0  After=0.5  SampleTime=0
  Step1 : Step  Time=0  After=0.5  SampleTime=0
  Subsystem : Subsystem
  Subsystem1 : Subsystem
  Subsystem2 : Subsystem
  Terminator : Terminator
  Uniform Random Number : UniformRandomNumber  Minimum=-0.5  Maximum=0.5  SampleTime=4
  Uniform Random Number1 : UniformRandomNumber  Minimum=-0.5  Maximum=0.5  Seed=6  SampleTime=7
  Unit Delay : UnitDelay  SampleTime=Tm  HasFrameUpgradeWarning=on
  wires:
  Gain/1 -> Add/2
  Mux/1 -> Add1/1
  [Ruido_actuador] -> Add/1
  Add6/1 -> Subsystem1/2(Y), Demux1/1
  Gain1/1 -> Add/3
  [Ruido_sensor] -> Add6/1
  Demux1/2 -> [Y2_nl]
  [Sp1] -> Mux/1
  [Y1_nl] -> Mux1/1
  Subsystem1/1(Estados) -> Demux6/1, Manual Switch2/2
  Mux1/1 -> Add1/2
  Add8/1 -> Gain/1, Unit Delay/1
  [Sp2] -> Mux/2
  [Sp1] -> Mux3/1
  [Sp2] -> Mux3/2
  Demux2/1 -> [Y1_l]
  [Y2_nl] -> Mux1/2
  Demux1/1 -> [Y1_nl]
  Demux2/2 -> [Y2_l]
  [Y1_l] -> Mux4/1
  [Y2_l] -> Mux4/2
  Manual Switch2/1 -> Gain1/1
  Add1/1 -> Add8/1
  Unit Delay/1 -> Add8/2
  Demux/2 -> Subsystem/2(In2)
  Demux/1 -> Subsystem/1(In1)
  Demux/3 -> Subsystem/3(In3)
  Add/1 -> Demux/1, Subsystem1/1(U), [U_nl]
  Subsystem/1(Y) -> Add6/2
  Subsystem/2(Est) -> Demux5/1, Manual Switch2/1
  Mux10/1 -> Scope5/3
  Mux9/1 -> Scope5/2
  Mux8/1 -> Scope5/1
  Demux5/2 -> Mux9/1
  Demux6/3 -> Mux10/2
  Demux5/3 -> Mux10/1
  Demux5/1 -> Mux8/1
  Demux6/2 -> Mux9/2
  Demux6/1 -> Mux8/2
  Demux3/2 -> Subsystem2/2(In2)
  Demux3/1 -> Subsystem2/1(In1)
  [Ruido_sensor] -> Add3/1
  Demux3/3 -> Subsystem2/3(In3)
  Subsystem2/1(Y) -> Add3/2
  [Ruido_actuador] -> Add2/1
  Add2/1 -> Demux3/1, [U_l]
  Mux3/1 -> Mux12/1
  Mux4/1 -> Mux12/2
  Mux12/1 -> Discrete State-Space/1
  Discrete State-Space/1 -> Add2/2
  Subsystem2/2(Est) -> Terminator/1
  Add3/1 -> Demux2/1
  [Sp2] -> Mux5/1  "Sp"
  Mux5/1 -> Scope/2
  [Y1_nl] -> Mux2/2  "NL"
  [Y1_l] -> Mux2/3  "L"
  Mux2/1 -> Scope/1
  [Y2_l] -> Mux5/3  "L"
  [Sp1] -> Mux2/1  "Sp"
  [U_l] -> Scope1/2
  [U_nl] -> Scope1/1
  [Y2_nl] -> Mux5/2  "NL"
  Manual Switch/1 -> [Sp1]
  Uniform Random Number/1 -> Manual Switch/2
  Uniform Random Number1/1 -> Manual Switch1/2
  Step/1 -> Manual Switch/1
  Step1/1 -> Manual Switch1/1
  Band-Limited White Noise1/1 -> [Ruido_sensor]
  Manual Switch1/1 -> [Sp2]
  Band-Limited White Noise/1 -> [Ruido_actuador]

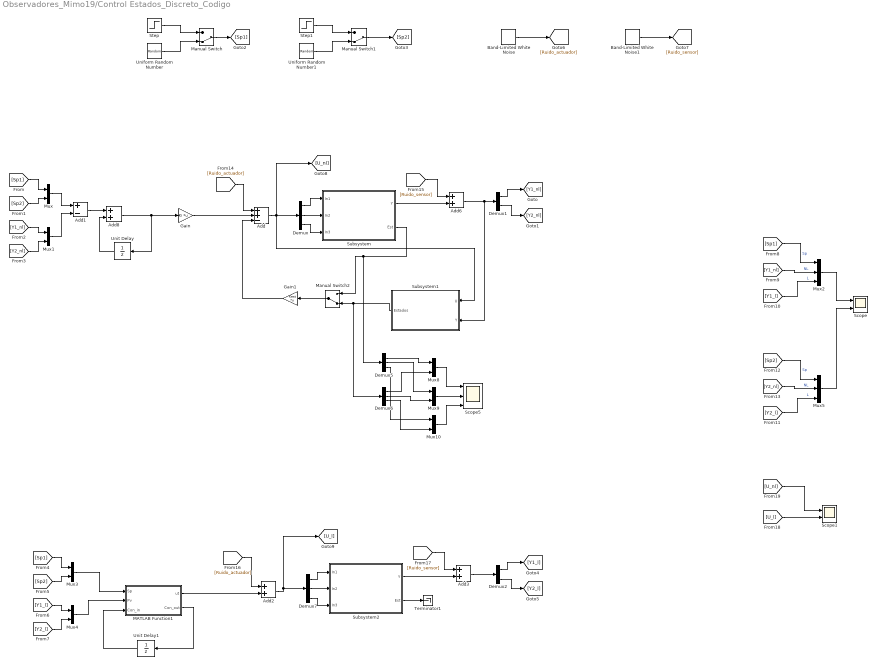
== system Observadores_Mimo19/Control Estados_Discreto_Codigo ==
  Add : Sum  Inputs=++-
  Add1 : Sum  Inputs=+-
  Add{2..3,6,8} (4 alike) : Sum
  Band-Limited White Noise : simulink/Sources/Band-Limited White Noise  Cov=[1e-10 1e-10 1e-10 ]  Ts=0.001  seed=[23341]
  Band-Limited White Noise1 : simulink/Sources/Band-Limited White Noise  Cov=[1e-10 1e-10 ]  Ts=0.001  seed=[23341]
  Demux{,5..7} (4 alike) : Demux  Outputs=3
  Demux1 : Demux  Outputs=2
  Demux2 : Demux  Outputs=2
  Gain : Gain  Gain=Ki  Multiplication=Matrix(K*u)
  Gain1 : Gain  Gain=Kest  Multiplication=Matrix(K*u)
  MATLAB Function1 : MATLAB Function  TreatAsAtomicUnit=on
  Manual Switch : ManualSwitch  CurrentSetting=0
  Manual Switch1 : ManualSwitch  CurrentSetting=0
  Manual Switch2 : ManualSwitch  CurrentSetting=0
  Mux{,1,3..4,8..10} (7 alike) : Mux  Inputs=2
  Mux2 : Mux  Inputs=3
  Mux5 : Mux  Inputs=3
  Scope : Scope  NumInputPorts=2
  Scope1 : Scope  NumInputPorts=2
  Scope5 : Scope  NumInputPorts=3
  Step : Step  Time=0  After=0.5  SampleTime=0
  Step1 : Step  Time=0  After=0.5  SampleTime=0
  Subsystem : Subsystem
  Subsystem1 : Subsystem
  Subsystem2 : Subsystem
  Terminator1 : Terminator
  Uniform Random Number : UniformRandomNumber  Minimum=-0.5  Maximum=0.5  SampleTime=4
  Uniform Random Number1 : UniformRandomNumber  Minimum=-0.5  Maximum=0.5  Seed=6  SampleTime=7
  Unit Delay : UnitDelay  SampleTime=Tm  HasFrameUpgradeWarning=on
  Unit Delay1 : UnitDelay  InitialCondition=zeros(8,1)  SampleTime=Tm  HasFrameUpgradeWarning=on
  wires:
  Gain/1 -> Add/2
  Mux/1 -> Add1/1
  [Ruido_actuador] -> Add/1
  Add6/1 -> Subsystem1/2(Y), Demux1/1
  Gain1/1 -> Add/3
  [Ruido_sensor] -> Add6/1
  Demux1/2 -> [Y2_nl]
  [Sp1] -> Mux/1
  [Y1_nl] -> Mux1/1
  Subsystem1/1(Estados) -> Demux6/1, Manual Switch2/2
  Mux1/1 -> Add1/2
  Add8/1 -> Gain/1, Unit Delay/1
  [Sp2] -> Mux/2
  [Y2_nl] -> Mux1/2
  Demux1/1 -> [Y1_nl]
  Manual Switch2/1 -> Gain1/1
  Add1/1 -> Add8/1
  Unit Delay/1 -> Add8/2
  Demux/2 -> Subsystem/2(In2)
  Demux/1 -> Subsystem/1(In1)
  Demux/3 -> Subsystem/3(In3)
  Add/1 -> Demux/1, Subsystem1/1(U), [U_nl]
  Subsystem/1(Y) -> Add6/2
  Subsystem/2(Est) -> Demux5/1, Manual Switch2/1
  Mux10/1 -> Scope5/3
  Mux9/1 -> Scope5/2
  Mux8/1 -> Scope5/1
  Demux5/2 -> Mux9/1
  Demux6/3 -> Mux10/2
  Demux5/3 -> Mux10/1
  Demux5/1 -> Mux8/1
  Demux6/2 -> Mux9/2
  Demux6/1 -> Mux8/2
  Add2/1 -> Demux7/1, [U_l]
  Demux7/3 -> Subsystem2/3(In3)
  Subsystem2/1(Y) -> Add3/2
  [Ruido_actuador] -> Add2/1
  Demux7/1 -> Subsystem2/1(In1)
  Demux7/2 -> Subsystem2/2(In2)
  Subsystem2/2(Est) -> Terminator1/1
  [Y1_l] -> Mux4/1
  [Sp2] -> Mux3/2
  [Y2_l] -> Mux4/2
  Demux2/2 -> [Y2_l]
  [Sp1] -> Mux3/1
  [Ruido_sensor] -> Add3/1
  Demux2/1 -> [Y1_l]
  Add3/1 -> Demux2/1
  Manual Switch/1 -> [Sp1]
  Uniform Random Number/1 -> Manual Switch/2
  Uniform Random Number1/1 -> Manual Switch1/2
  Step/1 -> Manual Switch/1
  Step1/1 -> Manual Switch1/1
  Band-Limited White Noise1/1 -> [Ruido_sensor]
  Manual Switch1/1 -> [Sp2]
  Band-Limited White Noise/1 -> [Ruido_actuador]
  [U_nl] -> Scope1/1
  [U_l] -> Scope1/2
  [Y1_nl] -> Mux2/2  "NL"
  [Sp1] -> Mux2/1  "Sp"
  [Y2_nl] -> Mux5/2  "NL"
  Mux2/1 -> Scope/1
  [Y1_l] -> Mux2/3  "L"
  [Y2_l] -> Mux5/3  "L"
  Mux5/1 -> Scope/2
  [Sp2] -> Mux5/1  "Sp"
  Unit Delay1/1 -> MATLAB Function1/3(Con_in)
  MATLAB Function1/2(Con_out) -> Unit Delay1/1
  MATLAB Function1/1(ut) -> Add2/2
  Mux3/1 -> MATLAB Function1/1(Sp)
  Mux4/1 -> MATLAB Function1/2(Pv)

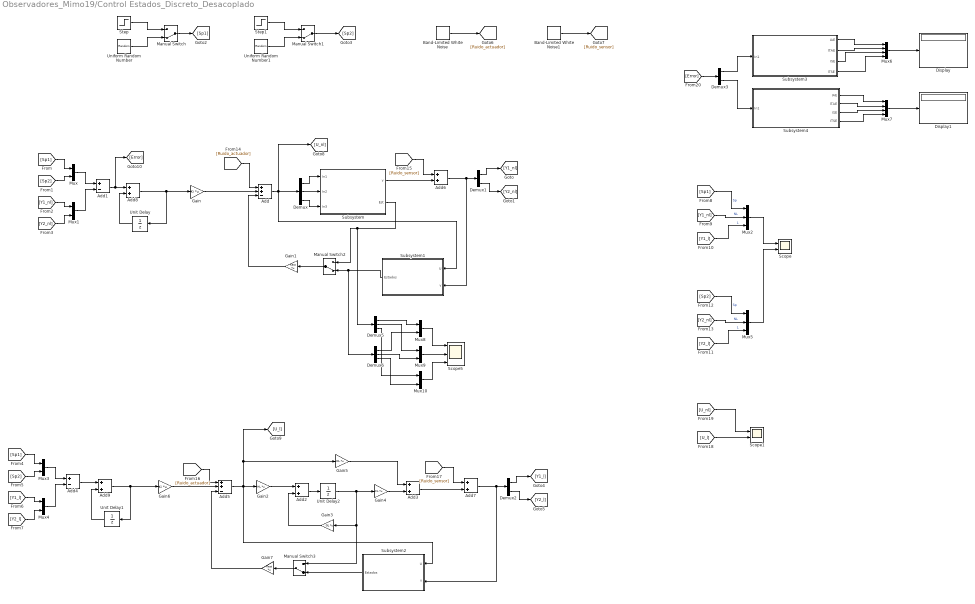
== system Observadores_Mimo19/Control Estados_Discreto_Desacoplado ==
  Add : Sum  Inputs=++-
  Add1 : Sum  Inputs=+-
  Add{2..3,6..9} (6 alike) : Sum
  Add4 : Sum  Inputs=+-
  Add5 : Sum  Inputs=++-
  Band-Limited White Noise : simulink/Sources/Band-Limited White Noise  Cov=[1e-10 1e-10 1e-10 ]  Ts=0.001  seed=[23341]
  Band-Limited White Noise1 : simulink/Sources/Band-Limited White Noise  Cov=[1e-10 1e-10 ]  Ts=0.001  seed=[23341]
  Demux : Demux  Outputs=3
  Demux1 : Demux  Outputs=2
  Demux2 : Demux  Outputs=2
  Demux3 : Demux  Outputs=2
  Demux5 : Demux  Outputs=3
  Demux6 : Demux  Outputs=3
  Display : Display
  Display1 : Display
  Gain : Gain  Gain=Ki  Multiplication=Matrix(K*u)
  Gain1 : Gain  Gain=Kest  Multiplication=Matrix(K*u)
  Gain2 : Gain  Gain=HL  Multiplication=Matrix(K*u)
  Gain3 : Gain  Gain=GL  Multiplication=Matrix(K*u)
  Gain4 : Gain  Gain=CL  Multiplication=Matrix(K*u)
  Gain5 : Gain  Gain=DL  Multiplication=Matrix(K*u)
  Gain6 : Gain  Gain=Ki  Multiplication=Matrix(K*u)
  Gain7 : Gain  Gain=Kest  Multiplication=Matrix(K*u)
  Manual Switch{,1..3} (4 alike) : ManualSwitch  CurrentSetting=0
  Mux{,1,3..4,8..10} (7 alike) : Mux  Inputs=2
  Mux2 : Mux  Inputs=3
  Mux5 : Mux  Inputs=3
  Mux6 : Mux
  Mux7 : Mux
  Scope : Scope  NumInputPorts=2
  Scope1 : Scope  NumInputPorts=2
  Scope5 : Scope  NumInputPorts=3
  Step : Step  Time=0  After=0.5  SampleTime=0
  Step1 : Step  Time=0  After=0.5  SampleTime=0
  Subsystem : Subsystem
  Subsystem1 : Subsystem
  Subsystem2 : Subsystem
  Subsystem3 : Subsystem
  Subsystem4 : Subsystem
  Uniform Random Number : UniformRandomNumber  Minimum=-0.5  Maximum=0.5  SampleTime=4
  Uniform Random Number1 : UniformRandomNumber  Minimum=-0.5  Maximum=0.5  Seed=6  SampleTime=7
  Unit Delay : UnitDelay  SampleTime=Tm  HasFrameUpgradeWarning=on
  Unit Delay1 : UnitDelay  SampleTime=Tm  HasFrameUpgradeWarning=on
  Unit Delay2 : UnitDelay  SampleTime=Tm  HasFrameUpgradeWarning=on
  wires:
  Gain/1 -> Add/2
  Subsystem2/1(Estados) -> Manual Switch3/2
  [Sp2] -> Mux5/1  "Sp"
  Add7/1 -> Subsystem2/2(Y), Demux2/1
  Mux/1 -> Add1/1
  [Ruido_actuador] -> Add/1
  Add6/1 -> Subsystem1/2(Y), Demux1/1
  [Y1_nl] -> Mux2/2  "NL"
  [U_nl] -> Scope1/1
  Gain1/1 -> Add/3
  Add5/1 -> Subsystem2/1(U), [U_l], Gain5/1, Gain2/1
  [Ruido_sensor] -> Add6/1
  Gain2/1 -> Add2/1
  Gain5/1 -> Add3/1
  [Ruido_actuador] -> Add5/1
  [Y2_nl] -> Mux5/2  "NL"
  Demux1/2 -> [Y2_nl]
  [Sp1] -> Mux/1
  [Y1_nl] -> Mux1/1
  Subsystem1/1(Estados) -> Demux6/1, Manual Switch2/2
  [U_l] -> Scope1/2
  Gain7/1 -> Add5/3
  [Y2_l] -> Mux5/3  "L"
  Manual Switch3/1 -> Gain7/1
  Mux1/1 -> Add1/2
  [Ruido_sensor] -> Add7/1
  Gain4/1 -> Add3/2
  Add8/1 -> Gain/1, Unit Delay/1
  Mux4/1 -> Add4/2
  [Sp2] -> Mux/2
  [Sp1] -> Mux3/1
  Unit Delay2/1 -> Gain4/1, Gain3/1, Manual Switch3/1
  [Sp2] -> Mux3/2
  Demux2/1 -> [Y1_l]
  Gain3/1 -> Add2/2
  [Y2_nl] -> Mux1/2
  Mux2/1 -> Scope/1
  Demux1/1 -> [Y1_nl]
  [Sp1] -> Mux2/1  "Sp"
  Demux2/2 -> [Y2_l]
  [Y1_l] -> Mux4/1
  Mux3/1 -> Add4/1
  [Y2_l] -> Mux4/2
  [Y1_l] -> Mux2/3  "L"
  Manual Switch2/1 -> Gain1/1
  Add2/1 -> Unit Delay2/1
  Mux5/1 -> Scope/2
  Add3/1 -> Add7/2
  Add1/1 -> [Error], Add8/1
  Unit Delay/1 -> Add8/2
  Unit Delay1/1 -> Add9/2
  Add9/1 -> Gain6/1, Unit Delay1/1
  Gain6/1 -> Add5/2
  Add4/1 -> Add9/1
  Manual Switch1/1 -> [Sp2]
  Step1/1 -> Manual Switch1/1
  Step/1 -> Manual Switch/1
  Manual Switch/1 -> [Sp1]
  Uniform Random Number1/1 -> Manual Switch1/2
  Band-Limited White Noise1/1 -> [Ruido_sensor]
  Band-Limited White Noise/1 -> [Ruido_actuador]
  Uniform Random Number/1 -> Manual Switch/2
  Demux/2 -> Subsystem/2(In2)
  Demux/1 -> Subsystem/1(In1)
  Demux/3 -> Subsystem/3(In3)
  Add/1 -> Demux/1, Subsystem1/1(U), [U_nl]
  Subsystem/1(Y) -> Add6/2
  Subsystem/2(Est) -> Demux5/1, Manual Switch2/1
  Mux10/1 -> Scope5/3
  Mux9/1 -> Scope5/2
  Mux8/1 -> Scope5/1
  Demux5/2 -> Mux9/1
  Demux6/3 -> Mux10/2
  Demux5/3 -> Mux10/1
  Demux5/1 -> Mux8/1
  Demux6/2 -> Mux9/2
  Demux6/1 -> Mux8/2
  Subsystem3/4(ITSE) -> Mux6/4
  [Error] -> Demux3/1
  Subsystem4/3(ISE) -> Mux7/3
  Subsystem4/4(ITSE) -> Mux7/4
  Subsystem4/2(ITAE) -> Mux7/2
  Subsystem4/1(IAE) -> Mux7/1
  Mux6/1 -> Display/1
  Subsystem3/2(ITAE) -> Mux6/2
  Subsystem3/1(IAE) -> Mux6/1
  Demux3/2 -> Subsystem4/1(In1)
  Demux3/1 -> Subsystem3/1(In1)
  Mux7/1 -> Display1/1
  Subsystem3/3(ISE) -> Mux6/3

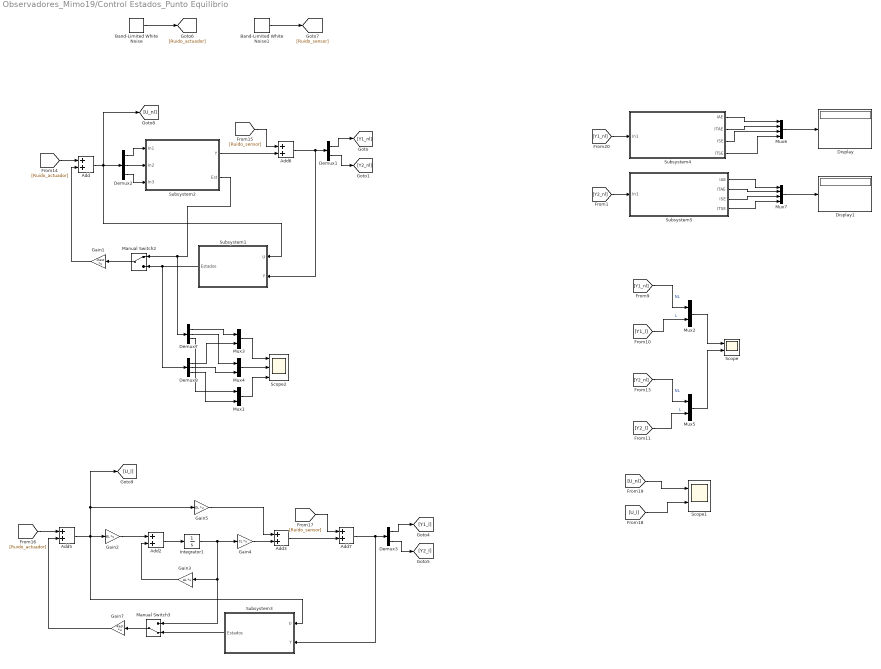
== system Observadores_Mimo19/Control Estados_Punto Equilibrio ==
  Add{,2..3,5..7} (6 alike) : Sum
  Band-Limited White Noise : simulink/Sources/Band-Limited White Noise  Cov=[1e-12 1e-12 1e-12 ]  Ts=0.001  seed=[23341]
  Band-Limited White Noise1 : simulink/Sources/Band-Limited White Noise  Cov=[1e-10 1e-10 ]  Ts=0.001  seed=[23341]
  Demux1 : Demux  Outputs=2
  Demux2 : Demux  Outputs=3
  Demux3 : Demux  Outputs=2
  Demux7 : Demux  Outputs=3
  Demux8 : Demux  Outputs=3
  Display : Display
  Display1 : Display
  Gain1 : Gain  Gain=-Kest  Multiplication=Matrix(K*u)
  Gain2 : Gain  Gain=BL  Multiplication=Matrix(K*u)
  Gain3 : Gain  Gain=AL  Multiplication=Matrix(K*u)
  Gain4 : Gain  Gain=CL  Multiplication=Matrix(K*u)
  Gain5 : Gain  Gain=DL  Multiplication=Matrix(K*u)
  Gain7 : Gain  Gain=-Kest  Multiplication=Matrix(K*u)
  Integrator1 : Integrator  InitialCondition=xini
  Manual Switch2 : ManualSwitch
  Manual Switch3 : ManualSwitch  CurrentSetting=0
  Mux{1..5} (5 alike) : Mux  Inputs=2
  Mux6 : Mux
  Mux7 : Mux
  Scope : Scope  NumInputPorts=2
  Scope1 : Scope  NumInputPorts=2
  Scope2 : Scope  NumInputPorts=3
  Subsystem1 : Subsystem
  Subsystem2 : Subsystem
  Subsystem3 : Subsystem
  Subsystem4 : Subsystem
  Subsystem5 : Subsystem
  wires:
  [U_nl] -> Scope1/1
  [U_l] -> Scope1/2
  Mux2/1 -> Scope/1
  Mux5/1 -> Scope/2
  [Y1_nl] -> Mux2/1  "NL"
  [Y1_l] -> Mux2/2  "L"
  [Y2_nl] -> Mux5/1  "NL"
  [Y2_l] -> Mux5/2  "L"
  Subsystem1/1(Estados) -> Demux8/1, Manual Switch2/2
  Demux1/1 -> [Y1_nl]
  Add6/1 -> Subsystem1/2(Y), Demux1/1
  [Ruido_actuador] -> Add/1
  Demux1/2 -> [Y2_nl]
  Add/1 -> Demux2/1, Subsystem1/1(U), [U_nl]
  Gain1/1 -> Add/2
  [Ruido_sensor] -> Add6/1
  Manual Switch2/1 -> Gain1/1
  Demux2/1 -> Subsystem2/1(In1)
  Demux2/2 -> Subsystem2/2(In2)
  Demux2/3 -> Subsystem2/3(In3)
  Subsystem2/1(Y) -> Add6/2
  Subsystem2/2(Est) -> Demux7/1, Manual Switch2/1
  Demux7/3 -> Mux1/1
  Demux8/1 -> Mux3/2
  Demux7/1 -> Mux3/1
  Mux1/1 -> Scope2/3
  Demux8/2 -> Mux4/2
  Mux4/1 -> Scope2/2
  Mux3/1 -> Scope2/1
  Demux8/3 -> Mux1/2
  Demux7/2 -> Mux4/1
  Add2/1 -> Integrator1/1
  [Ruido_actuador] -> Add5/1
  Subsystem3/1(Estados) -> Manual Switch3/2
  Gain7/1 -> Add5/2
  Demux3/2 -> [Y2_l]
  Add3/1 -> Add7/2
  Demux3/1 -> [Y1_l]
  Add5/1 -> Subsystem3/1(U), [U_l], Gain5/1, Gain2/1
  Gain4/1 -> Add3/2
  Gain5/1 -> Add3/1
  Integrator1/1 -> Gain4/1, Gain3/1, Manual Switch3/1
  Gain3/1 -> Add2/2
  Manual Switch3/1 -> Gain7/1
  Add7/1 -> Subsystem3/2(Y), Demux3/1
  [Ruido_sensor] -> Add7/1
  Gain2/1 -> Add2/1
  Band-Limited White Noise/1 -> [Ruido_actuador]
  Band-Limited White Noise1/1 -> [Ruido_sensor]
  Subsystem4/4(ITSE) -> Mux6/4
  Subsystem5/3(ISE) -> Mux7/3
  Subsystem5/4(ITSE) -> Mux7/4
  Subsystem5/2(ITAE) -> Mux7/2
  Subsystem5/1(IAE) -> Mux7/1
  Mux6/1 -> Display/1
  Subsystem4/2(ITAE) -> Mux6/2
  Subsystem4/1(IAE) -> Mux6/1
  Mux7/1 -> Display1/1
  Subsystem4/3(ISE) -> Mux6/3
  [Y1_nl] -> Subsystem4/1(In1)
  [Y2_nl] -> Subsystem5/1(In1)

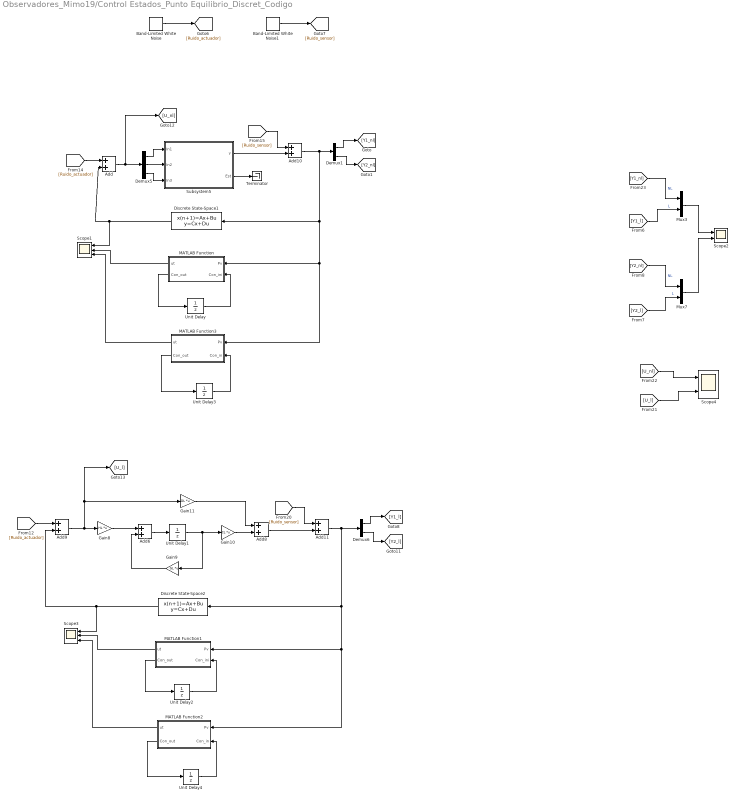
== system Observadores_Mimo19/Control Estados_Punto Equilibrio_Discret_Codigo ==
  Add{,6,8..11} (6 alike) : Sum
  Band-Limited White Noise : simulink/Sources/Band-Limited White Noise  Cov=[1e-12 1e-12 1e-12 ]  Ts=0.001  seed=[23341]
  Band-Limited White Noise1 : simulink/Sources/Band-Limited White Noise  Cov=[1e-10 1e-10 ]  Ts=0.001  seed=[23341]
  Demux1 : Demux  Outputs=2
  Demux5 : Demux  Outputs=3
  Demux6 : Demux  Outputs=2
  Discrete State-Space1 : DiscreteStateSpace  A=Gc  B=Hc  C=Cc  D=Dc  SampleTime=Tm
  Discrete State-Space2 : DiscreteStateSpace  A=Gc  B=Hc  C=Cc  D=Dc  SampleTime=Tm
  Gain10 : Gain  Gain=CL  Multiplication=Matrix(K*u)
  Gain11 : Gain  Gain=DL  Multiplication=Matrix(K*u)
  Gain8 : Gain  Gain=HL  Multiplication=Matrix(K*u)
  Gain9 : Gain  Gain=GL  Multiplication=Matrix(K*u)
  MATLAB Function : MATLAB Function  TreatAsAtomicUnit=on
  MATLAB Function1 : MATLAB Function  TreatAsAtomicUnit=on
  MATLAB Function2 : MATLAB Function  TreatAsAtomicUnit=on
  MATLAB Function3 : MATLAB Function  TreatAsAtomicUnit=on
  Mux3 : Mux  Inputs=2
  Mux7 : Mux  Inputs=2
  Scope1 : Scope  NumInputPorts=3
  Scope2 : Scope  NumInputPorts=2
  Scope3 : Scope  NumInputPorts=3
  Scope4 : Scope  NumInputPorts=2
  Subsystem5 : Subsystem
  Terminator : Terminator
  Unit Delay{,2..4} (4 alike) : UnitDelay  InitialCondition=zeros(3,1)  SampleTime=Tm  HasFrameUpgradeWarning=on
  Unit Delay1 : UnitDelay  InitialCondition=xini  SampleTime=Tm  HasFrameUpgradeWarning=on
  wires:
  [Y1_nl] -> Mux3/1  "NL"
  Mux3/1 -> Scope2/1
  Mux7/1 -> Scope2/2
  [Y2_nl] -> Mux7/1  "NL"
  [U_l] -> Scope4/2
  [U_nl] -> Scope4/1
  Demux5/2 -> Subsystem5/2(In2)
  Gain8/1 -> Add6/1
  [Y2_l] -> Mux7/2  "L"
  [Ruido_sensor] -> Add11/1
  Subsystem5/1(Y) -> Add10/2
  Add9/1 -> [U_l], Gain11/1, Gain8/1
  Gain11/1 -> Add8/1
  Gain10/1 -> Add8/2
  Demux6/2 -> [Y2_l]
  Add8/1 -> Add11/2
  Add6/1 -> Unit Delay1/1
  [Ruido_actuador] -> Add9/1
  [Y1_l] -> Mux3/2  "L"
  Unit Delay1/1 -> Gain10/1, Gain9/1
  Demux5/1 -> Subsystem5/1(In1)
  [Ruido_sensor] -> Add10/1
  Demux6/1 -> [Y1_l]
  [Ruido_actuador] -> Add/1
  Add/1 -> Demux5/1, [U_nl]
  Demux1/2 -> [Y2_nl]
  Gain9/1 -> Add6/2
  Demux1/1 -> [Y1_nl]
  Demux5/3 -> Subsystem5/3(In3)
  Subsystem5/2(Est) -> Terminator/1
  Add10/1 -> MATLAB Function3/1(Pv), MATLAB Function/1(Pv), Discrete State-Space1/1, Demux1/1
  Band-Limited White Noise1/1 -> [Ruido_sensor]
  Band-Limited White Noise/1 -> [Ruido_actuador]
  MATLAB Function/2(Con_out) -> Unit Delay/1
  Unit Delay3/1 -> MATLAB Function3/2(Con_in)
  MATLAB Function/1(ut) -> Scope1/2
  MATLAB Function3/1(ut) -> Scope1/3
  MATLAB Function3/2(Con_out) -> Unit Delay3/1
  Unit Delay/1 -> MATLAB Function/2(Con_ini)
  Discrete State-Space1/1 -> Scope1/1, Add/2
  MATLAB Function1/1(ut) -> Scope3/2
  Unit Delay2/1 -> MATLAB Function1/2(Con_ini)
  MATLAB Function2/2(Con_out) -> Unit Delay4/1
  MATLAB Function1/2(Con_out) -> Unit Delay2/1
  MATLAB Function2/1(ut) -> Scope3/3
  Discrete State-Space2/1 -> Add9/2, Scope3/1
  Unit Delay4/1 -> MATLAB Function2/2(Con_in)
  Add11/1 -> MATLAB Function2/1(Pv), MATLAB Function1/1(Pv), Discrete State-Space2/1, Demux6/1

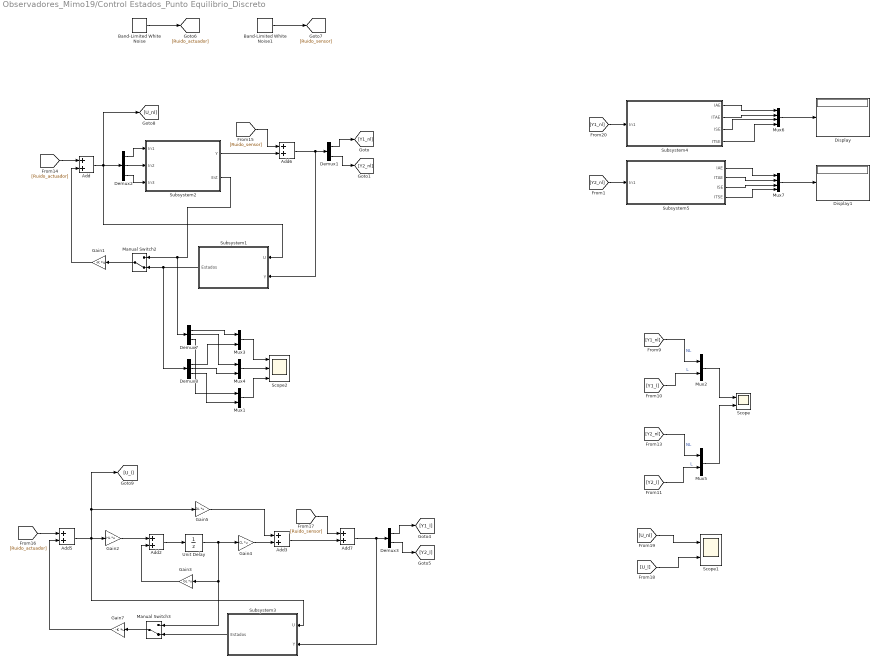
== system Observadores_Mimo19/Control Estados_Punto Equilibrio_Discreto ==
  Add{,2..3,5..7} (6 alike) : Sum
  Band-Limited White Noise : simulink/Sources/Band-Limited White Noise  Cov=[1e-12 1e-12 1e-12 ]  Ts=0.001  seed=[23341]
  Band-Limited White Noise1 : simulink/Sources/Band-Limited White Noise  Cov=[1e-10 1e-10 ]  Ts=0.001  seed=[23341]
  Demux1 : Demux  Outputs=2
  Demux2 : Demux  Outputs=3
  Demux3 : Demux  Outputs=2
  Demux7 : Demux  Outputs=3
  Demux8 : Demux  Outputs=3
  Display : Display
  Display1 : Display
  Gain1 : Gain  Gain=-K  Multiplication=Matrix(K*u)
  Gain2 : Gain  Gain=HL  Multiplication=Matrix(K*u)
  Gain3 : Gain  Gain=GL  Multiplication=Matrix(K*u)
  Gain4 : Gain  Gain=CL  Multiplication=Matrix(K*u)
  Gain5 : Gain  Gain=DL  Multiplication=Matrix(K*u)
  Gain7 : Gain  Gain=-K  Multiplication=Matrix(K*u)
  Manual Switch2 : ManualSwitch  CurrentSetting=0
  Manual Switch3 : ManualSwitch  CurrentSetting=0
  Mux{1..5} (5 alike) : Mux  Inputs=2
  Mux6 : Mux
  Mux7 : Mux
  Scope : Scope  NumInputPorts=2
  Scope1 : Scope  NumInputPorts=2
  Scope2 : Scope  NumInputPorts=3
  Subsystem1 : Subsystem
  Subsystem2 : Subsystem
  Subsystem3 : Subsystem
  Subsystem4 : Subsystem
  Subsystem5 : Subsystem
  Unit Delay : UnitDelay  SampleTime=Tm  HasFrameUpgradeWarning=on
  wires:
  [U_nl] -> Scope1/1
  [U_l] -> Scope1/2
  Mux2/1 -> Scope/1
  Mux5/1 -> Scope/2
  [Y1_nl] -> Mux2/1  "NL"
  [Y1_l] -> Mux2/2  "L"
  [Y2_nl] -> Mux5/1  "NL"
  [Y2_l] -> Mux5/2  "L"
  Subsystem1/1(Estados) -> Demux8/1, Manual Switch2/2
  Demux1/1 -> [Y1_nl]
  Add6/1 -> Subsystem1/2(Y), Demux1/1
  [Ruido_actuador] -> Add/1
  Demux1/2 -> [Y2_nl]
  Add/1 -> Demux2/1, Subsystem1/1(U), [U_nl]
  Gain1/1 -> Add/2
  [Ruido_sensor] -> Add6/1
  Manual Switch2/1 -> Gain1/1
  Demux2/1 -> Subsystem2/1(In1)
  Demux2/2 -> Subsystem2/2(In2)
  Demux2/3 -> Subsystem2/3(In3)
  Subsystem2/1(Y) -> Add6/2
  Subsystem2/2(Est) -> Demux7/1, Manual Switch2/1
  Demux7/3 -> Mux1/1
  Demux8/1 -> Mux3/2
  Demux7/1 -> Mux3/1
  Mux1/1 -> Scope2/3
  Demux8/2 -> Mux4/2
  Mux4/1 -> Scope2/2
  Mux3/1 -> Scope2/1
  Demux8/3 -> Mux1/2
  Demux7/2 -> Mux4/1
  Add2/1 -> Unit Delay/1
  [Ruido_actuador] -> Add5/1
  Subsystem3/1(Estados) -> Manual Switch3/2
  Gain7/1 -> Add5/2
  Demux3/2 -> [Y2_l]
  Add3/1 -> Add7/2
  Demux3/1 -> [Y1_l]
  Add5/1 -> Subsystem3/1(U), [U_l], Gain5/1, Gain2/1
  Gain4/1 -> Add3/2
  Gain5/1 -> Add3/1
  Unit Delay/1 -> Gain3/1, Manual Switch3/1, Gain4/1
  Gain3/1 -> Add2/2
  Manual Switch3/1 -> Gain7/1
  Add7/1 -> Subsystem3/2(Y), Demux3/1
  [Ruido_sensor] -> Add7/1
  Gain2/1 -> Add2/1
  Band-Limited White Noise/1 -> [Ruido_actuador]
  Band-Limited White Noise1/1 -> [Ruido_sensor]
  Subsystem4/3(ISE) -> Mux6/3
  Subsystem4/1(IAE) -> Mux6/1
  Subsystem5/1(IAE) -> Mux7/1
  Subsystem4/2(ITAE) -> Mux6/2
  Mux6/1 -> Display/1
  Subsystem5/2(ITAE) -> Mux7/2
  Subsystem5/4(ITSE) -> Mux7/4
  Subsystem5/3(ISE) -> Mux7/3
  Subsystem4/4(ITSE) -> Mux6/4
  Mux7/1 -> Display1/1
  [Y1_nl] -> Subsystem4/1(In1)
  [Y2_nl] -> Subsystem5/1(In1)

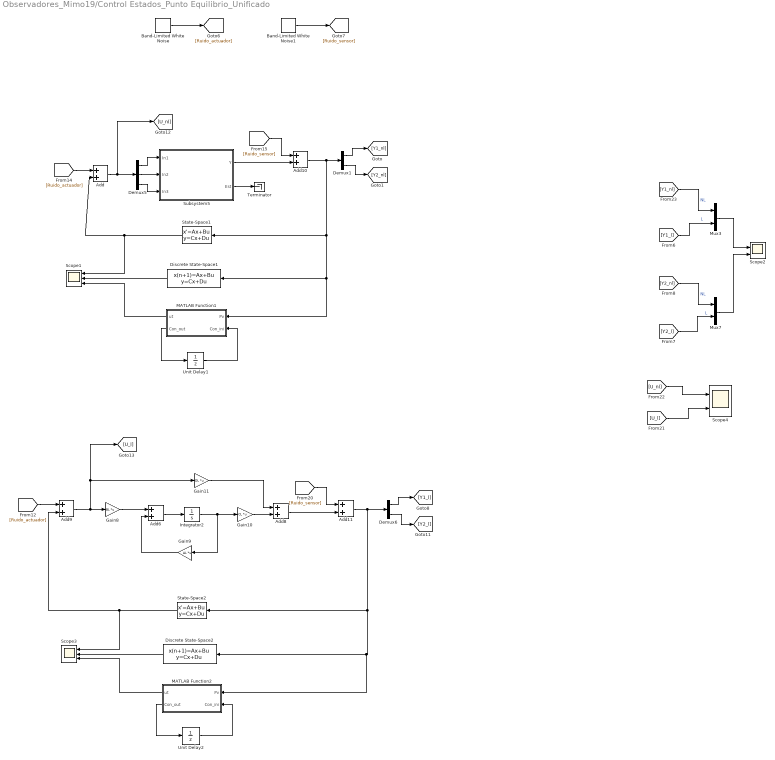
== system Observadores_Mimo19/Control Estados_Punto Equilibrio_Unificado ==
  Add{,6,8..11} (6 alike) : Sum
  Band-Limited White Noise : simulink/Sources/Band-Limited White Noise  Cov=[1e-12 1e-12 1e-12 ]  Ts=0.001  seed=[23341]
  Band-Limited White Noise1 : simulink/Sources/Band-Limited White Noise  Cov=[1e-10 1e-10 ]  Ts=0.001  seed=[23341]
  Demux1 : Demux  Outputs=2
  Demux5 : Demux  Outputs=3
  Demux6 : Demux  Outputs=2
  Discrete State-Space1 : DiscreteStateSpace  A=Gc  B=Hc  C=Cc  D=Dc  SampleTime=Tm
  Discrete State-Space2 : DiscreteStateSpace  A=Gc  B=Hc  C=Cc  D=Dc  SampleTime=Tm
  Gain10 : Gain  Gain=CL  Multiplication=Matrix(K*u)
  Gain11 : Gain  Gain=DL  Multiplication=Matrix(K*u)
  Gain8 : Gain  Gain=BL  Multiplication=Matrix(K*u)
  Gain9 : Gain  Gain=AL  Multiplication=Matrix(K*u)
  Integrator2 : Integrator  InitialCondition=xini
  MATLAB Function1 : MATLAB Function  TreatAsAtomicUnit=on
  MATLAB Function2 : MATLAB Function  TreatAsAtomicUnit=on
  Mux3 : Mux  Inputs=2
  Mux7 : Mux  Inputs=2
  Scope1 : Scope  NumInputPorts=3
  Scope2 : Scope  NumInputPorts=2
  Scope3 : Scope  NumInputPorts=3
  Scope4 : Scope  NumInputPorts=2
  State-Space1 : StateSpace  A=Ac  B=Bc  C=Cc  D=Dc  InitialCondition=0
  State-Space2 : StateSpace  A=Ac  B=Bc  C=Cc  D=Dc  InitialCondition=0
  Subsystem5 : Subsystem
  Terminator : Terminator
  Unit Delay1 : UnitDelay  InitialCondition=zeros(3,1)  SampleTime=Tm  HasFrameUpgradeWarning=on
  Unit Delay2 : UnitDelay  InitialCondition=zeros(3,1)  SampleTime=Tm  HasFrameUpgradeWarning=on
  wires:
  [Y1_nl] -> Mux3/1  "NL"
  Mux3/1 -> Scope2/1
  Mux7/1 -> Scope2/2
  [Y2_nl] -> Mux7/1  "NL"
  [U_l] -> Scope4/2
  [U_nl] -> Scope4/1
  Demux5/2 -> Subsystem5/2(In2)
  Gain8/1 -> Add6/1
  [Y2_l] -> Mux7/2  "L"
  [Ruido_sensor] -> Add11/1
  Subsystem5/1(Y) -> Add10/2
  Add9/1 -> [U_l], Gain11/1, Gain8/1
  Gain11/1 -> Add8/1
  Gain10/1 -> Add8/2
  Demux6/2 -> [Y2_l]
  Add8/1 -> Add11/2
  Add6/1 -> Integrator2/1
  [Ruido_actuador] -> Add9/1
  [Y1_l] -> Mux3/2  "L"
  Integrator2/1 -> Gain10/1, Gain9/1
  Demux5/1 -> Subsystem5/1(In1)
  [Ruido_sensor] -> Add10/1
  Demux6/1 -> [Y1_l]
  [Ruido_actuador] -> Add/1
  Add/1 -> Demux5/1, [U_nl]
  Demux1/2 -> [Y2_nl]
  Gain9/1 -> Add6/2
  Demux1/1 -> [Y1_nl]
  Demux5/3 -> Subsystem5/3(In3)
  Subsystem5/2(Est) -> Terminator/1
  Add10/1 -> MATLAB Function1/1(Pv), Discrete State-Space1/1, State-Space1/1, Demux1/1
  Unit Delay1/1 -> MATLAB Function1/2(Con_ini)
  MATLAB Function1/2(Con_out) -> Unit Delay1/1
  State-Space1/1 -> Add/2, Scope1/1
  Discrete State-Space1/1 -> Scope1/2
  MATLAB Function1/1(ut) -> Scope1/3
  State-Space2/1 -> Add9/2, Scope3/1
  MATLAB Function2/2(Con_out) -> Unit Delay2/1
  Discrete State-Space2/1 -> Scope3/2
  Unit Delay2/1 -> MATLAB Function2/2(Con_ini)
  Add11/1 -> MATLAB Function2/1(Pv), Discrete State-Space2/1, State-Space2/1, Demux6/1
  MATLAB Function2/1(ut) -> Scope3/3
  Band-Limited White Noise/1 -> [Ruido_actuador]
  Band-Limited White Noise1/1 -> [Ruido_sensor]

== system Observadores_Mimo19/Comparacion/Subsystem ==
  In1 : Inport
  In2 : Inport  Port=2
  In3 : Inport  Port=3
  Add : Sum
  Add1 : Sum
  Add2 : Sum
  Add4 : Sum  Inputs=+-
  Constant : Constant  Value=u10
  Constant1 : Constant  Value=u20
  Constant2 : Constant  Value=u30
  Constant4 : Constant  Value=[x10; x20; x30]
  Gain : Gain  Gain=CL  Multiplication=Matrix(K*u)
  Integrator : Integrator  InitialCondition=[x10; x20; x30]
  MATLAB Function : MATLAB Function  TreatAsAtomicUnit=on
  Y : Outport  VectorParamsAs1DForOutWhenUnconnected=off
  Est : Outport  Port=2  VectorParamsAs1DForOutWhenUnconnected=off
  wires:
  Constant1/1 -> Add1/1
  Add4/1 -> Est/1, Gain/1
  In2/1 -> Add1/2
  Constant/1 -> Add/1
  In1/1 -> Add/2
  Gain/1 -> Y/1
  Integrator/1 -> MATLAB Function/1(x), Add4/1
  Constant4/1 -> Add4/2
  In3/1 -> Add2/2
  Constant2/1 -> Add2/1
  Add/1 -> MATLAB Function/2(u1)
  MATLAB Function/1(f) -> Integrator/1
  Add1/1 -> MATLAB Function/3(u2)
  Add2/1 -> MATLAB Function/4(u3)

== system Observadores_Mimo19/Comparacion/Subsystem1 ==
  In1 : Inport
  In2 : Inport  Port=2
  In3 : Inport  Port=3
  Add : Sum
  Add1 : Sum
  Add2 : Sum
  Add4 : Sum  Inputs=+-
  Constant : Constant  Value=u10
  Constant1 : Constant  Value=u20
  Constant2 : Constant  Value=u30
  Constant4 : Constant  Value=[x10; x20; x30]
  Gain : Gain  Gain=CL  Multiplication=Matrix(K*u)
  Integrator : Integrator  InitialCondition=[x10; x20; x30]
  MATLAB Function : MATLAB Function  TreatAsAtomicUnit=on
  Y : Outport  VectorParamsAs1DForOutWhenUnconnected=off
  Est : Outport  Port=2  VectorParamsAs1DForOutWhenUnconnected=off
  wires:
  Constant1/1 -> Add1/1
  Add4/1 -> Est/1, Gain/1
  In2/1 -> Add1/2
  Constant/1 -> Add/1
  In1/1 -> Add/2
  Gain/1 -> Y/1
  Integrator/1 -> MATLAB Function/1(x), Add4/1
  Constant4/1 -> Add4/2
  In3/1 -> Add2/2
  Constant2/1 -> Add2/1
  Add/1 -> MATLAB Function/2(u1)
  MATLAB Function/1(f) -> Integrator/1
  Add1/1 -> MATLAB Function/3(u2)
  Add2/1 -> MATLAB Function/4(u3)
